simulink model "benchmark_model_2"  (R2021a)
settings: Solver=ode1  StartTime=0.0  StopTime=Tend  FixedStep=0.0001  MaxStep=0.1  MinStep=0.0001  AbsTol=0.01  EnableMultiTasking=on
values from neighbouring files (symbols this model uses):
  A1 = 0.00017774967488    [engine_data.mat]
  A2 = 740220.330082    [engine_data.mat]
  AL = [6 6.5 7 7.5 8 8.5 9 9.5 10 10.5 11 11.5 ... (33 elements, 33x1)]    [engine_data.mat]
  AM0 = 0.02884    [engine_data.mat]
  AREA = 0.00580880481649    [engine_data.mat]
  BORE = 0.086    [engine_data.mat]
  C_EGR = 1.5    [engine_data.mat]
  c_f = 800000    [engine_data.mat]
  c_T = 1    [engine_data.mat]
  CAIR = [0 0 0 0.21 0 0 0.79]    [engine_data.mat]
  cCO = 0    [engine_data.mat]
  cCO2 = 0    [engine_data.mat]
  cH2 = 0    [engine_data.mat]
  cH2O = 0    [engine_data.mat]
  cHC = 0    [engine_data.mat]
  cN2 = 0.79    [engine_data.mat]
  CO = [22.3416398376 20.8398063107 19.3759939408 17.9445472871 16.538827802 15.1528221174 13.7819470707 12.4234138404 11.076283262 9.74128071245 8.42044156849 7.11667724438 ... (33 elements, 33x1)]    [engine_data.mat]
  CO2 = [1.08016197936 1.63070203699 2.20578946805 2.80905596198 3.44329822989 4.11013545224 4.80975559522 5.54078746844 6.30033629562 7.08419123341 7.88717005398 8.70352822078 ... (33 elements, 33x1)]    [engine_data.mat]
  cO2 = 0.21    [engine_data.mat]
  DEN0 = 1.17881164668    [engine_data.mat]
  EGR_dia = 0.02    [engine_data.mat]
  EGR_sk = 0.125663706144    [engine_data.mat]
  EX_AREA = 0.00137444678595    [engine_data.mat]
  EX_M_AR = 0.0258532162804    [engine_data.mat]
  EXO = 40    [engine_data.mat]
  FD0 = 5    [engine_data.mat]
  FOM = [12 11.348 6.233 5 5.449 8.523 5]    [engine_data.mat]
  FR0 = 0    [engine_data.mat]
  FR_C1 = 305.731    [engine_data.mat]
  FR_C2 = 1.70183    [engine_data.mat]
  FR_C3 = 3188.7424    [engine_data.mat]
  FR_C4 = 0.000296028194151    [engine_data.mat]
  FR_C5 = 1.03    [engine_data.mat]
  H2 = [17.3855302766 15.0102176452 12.8820660449 10.9850020715 9.30240027035 7.81790027685 6.51548255669 5.37933989743 4.39378660966 3.5433012035 2.8127075229 2.1874445405 ... (33 elements, 33x1)]    [engine_data.mat]
  H2O = [3.81120036781 5.32559240945 6.64944794012 7.79700886885 8.78142378855 9.61507632366 10.310008356 10.8782622871 11.3320540899 11.6837509075 11.9456809954 12.1298414055 ... (33 elements, 33x1)]    [engine_data.mat]
  HC = [5481.3024964 4476.06435729 3754.34247414 3215.30411383 2799.83726136 2471.30975971 2205.97110777 1987.83348465 1805.78690133 1651.89669698 1520.35918152 1406.8402103 ... (33 elements, 33x1)]    [engine_data.mat]
  INC = 0    [engine_data.mat]
  INO = -40    [engine_data.mat]
  KET = 0.001    [engine_data.mat]
  Kex = 1.28224854645    [engine_data.mat]
  Kh = 0.00462    [engine_data.mat]
  MAS0 = 0.00471524658673    [engine_data.mat]
  MCh = 0.000588883862304    [engine_data.mat]
  MHC = 0.01383448    [engine_data.mat]
  MN2 = 0.028    [engine_data.mat]
  MO2 = 0.032    [engine_data.mat]
  MOLcylT = 0.00157069204711    [engine_data.mat]
  N2 = [54.5020363032 56.4529864816 58.2465252261 59.8999246568 61.4284172656 62.8453054261 64.1621746691 65.3891205654 66.5349581592 67.6074047194 68.6132342687 69.5584035698 ... (33 elements, 33x1)]    [engine_data.mat]
  O2 = [0.331300985803 0.293088680307 0.264743132617 0.242930742419 0.225648917415 0.211629427842 0.200034641439 0.190292592782 0.182002893523 0.174881554044 0.168729672297 0.163420998081 ... (33 elements, 33x1)]    [engine_data.mat]
  PR0 = 101324.72    [engine_data.mat]
  R150 = 157.079632679    [engine_data.mat]
  Rabs = 8.31441    [engine_data.mat]
  SPEC = [4 0.086 0.086 0.043 0.14665 14 1 0.1 0 0.5 0.005 0 ... (19 elements, 19x1)]    [engine_data.mat]
  TBORE = 0.055    [engine_data.mat]
  Tend = 120    [engine_data.mat]
  Th_HC = 0.1    [engine_data.mat]
  Th_knock = 0.401961937891    [engine_data.mat]
  THEX = [0 1 2 3 4 5 6 7 8 9 10 11 ... (721 elements, 1x721)]    [engine_data.mat]
  THIN = [0 1 2 3 4 5 6 7 8 9 10 11 ... (721 elements, 1x721)]    [engine_data.mat]
  TM0 = 298.15    [engine_data.mat]
  Tstart = 5    [engine_data.mat]
  TW0 = 353.15    [engine_data.mat]
  V_EX = 0.0001    [engine_data.mat]
  VAREX = [0 0 0 0 0 0 0 0 0 0 0 0 ... (721 elements, 1x721)]    [engine_data.mat]
  VARIN = [0 0 0 0 0 0 0 0 0 0 0 0 ... (721 elements, 1x721)]    [engine_data.mat]
  VH = 0.000499557214218    [engine_data.mat]
  VT = 3.84274780168e-05    [engine_data.mat]
  WOM = [0.01383448 0.04401 0.02801 0.032 0.002016 0.018016 0.028]    [engine_data.mat]
  y = 1.81    [engine_data.mat]
undefined symbols (not defined in the file or in its folder): DiscIntNeverNeededParam
libraries: pid_lib x3
(part 5 of 7)

== system benchmark_model_2/ENGINE/engine_s/cylinders/cyl3/cyl/knock_Integral/Subsystem1 ==
  pc : Inport
  rps : Inport  Port=2
  Tc : Inport  Port=3
  rad : Inport  Port=4
  Constant1 : Constant  Value=0
  Constant2 : Constant  Value=FR_C1
  Constant3 : Constant
  Constant4 : Constant  Value=(540+INC)*pi/180
  Constant5 : Constant  Value=(180-EXO)*pi/180
  Divide1 : Product  Inputs=3
  Divide2 : Product  Inputs=*/
  Fcn : Fcn  Expr=-FR_C2*(-FR_C4*u+FR_C5)
  Gain : Gain  Gain=0.001
  Integrator : Integrator  ExternalReset=rising
  Math Function : Math  Operator=pow  SignedPower=on  SaturateOnIntegerOverflow=on
  Memory : Memory
  Relational Operator1 : RelationalOperator  Operator=<=  OutDataTypeStr=boolean  RndMeth=Nearest
  Relational Operator2 : RelationalOperator  OutDataTypeStr=boolean  RndMeth=Nearest
  Saturation : Saturate  UpperLimit=inf  LowerLimit=1.0e-16
  Subsystem : Subsystem
  Switch : Switch  Threshold=0.5
  cal_unburned_temp : Subsystem
  ki : Outport
  wires:
  pc/1 -> Saturation/1
  Fcn/1 -> Math Function/2
  Math Function/1 -> Divide1/2
  Constant2/1 -> Divide1/1
  Subsystem/1(Out1) -> Divide1/3
  Divide1/1 -> Divide2/2
  Constant3/1 -> Divide2/1
  Divide2/1 -> Integrator/1
  Tc/1 -> cal_unburned_temp/2(Tc)
  Memory/1 -> Integrator/2
  cal_unburned_temp/1(Tu) -> Subsystem/1(Tu)
  Gain/1 -> Math Function/1
  Integrator/1 -> Switch/1
  Switch/1 -> ki/1
  Constant1/1 -> Switch/3
  rad/1 -> Relational Operator1/1, Relational Operator2/1
  Constant4/1 -> Relational Operator2/2
  Relational Operator2/1 -> cal_unburned_temp/3(trg_inc), Memory/1
  Constant5/1 -> Relational Operator1/2
  Relational Operator1/1 -> Switch/2
  rps/1 -> Fcn/1
  Saturation/1 -> cal_unburned_temp/1(Pc), Gain/1

== system benchmark_model_2/ENGINE/engine_s/cylinders/cyl3/cyl/knock_Integral/Triggered Subsystem ==
  QA_max : Inport
  QA : Inport  Port=2
  Trigger : TriggerPort  VariantControl=(inherit)
  Constant1 : Constant  Value=0
  Constant2 : Constant  Value=1.0e-9
  Relational Operator : RelationalOperator  OutDataTypeStr=boolean  RndMeth=Nearest
  Subtract : Sum  Inputs=+-
  Switch : Switch  Threshold=0.5
  AI_Q : Outport  InitialOutput=0
  wires:
  QA/1 -> Subtract/2
  QA_max/1 -> Subtract/1
  Constant1/1 -> Switch/3
  Switch/1 -> AI_Q/1
  Subtract/1 -> Relational Operator/1, Switch/1
  Relational Operator/1 -> Switch/2
  Constant2/1 -> Relational Operator/2

== system benchmark_model_2/ENGINE/engine_s/cylinders/cyl3/cyl/ramining ratio of fuel/Triggered Subsystem ==
  QA : Inport
  Trigger : TriggerPort  VariantControl=(inherit)
  Constant : Constant
  Constant1 : Constant  Value=0
  Constant2 : Constant  Value=1.0e-9
  Relational Operator : RelationalOperator  OutDataTypeStr=boolean  RndMeth=Nearest
  Subtract : Sum  Inputs=+-
  Switch : Switch  Threshold=0.5
  AI_Q : Outport  InitialOutput=0
  wires:
  Constant2/1 -> Relational Operator/2
  Relational Operator/1 -> Switch/2
  Subtract/1 -> Switch/1, Relational Operator/1
  Switch/1 -> AI_Q/1
  Constant1/1 -> Switch/3
  Constant/1 -> Subtract/1
  QA/1 -> Subtract/2

== system benchmark_model_2/ENGINE/engine_s/cylinders/cyl3/cyl/unburnt_gass/add_fuel1 ==
  Nfuel : Inport
  mol : Inport  Port=2
  Add : Sum
  Demux : Demux  Outputs=7
  Mux : Mux  Inputs=7
  add_fuel : Outport
  wires:
  Demux/2 -> Mux/2
  Demux/3 -> Mux/3
  Demux/4 -> Mux/4
  Demux/5 -> Mux/5
  Demux/6 -> Mux/6
  Demux/7 -> Mux/7
  mol/1 -> Demux/1
  Mux/1 -> add_fuel/1
  Demux/1 -> Add/2
  Add/1 -> Mux/1
  Nfuel/1 -> Add/1

== system benchmark_model_2/ENGINE/engine_s/cylinders/cyl3/cyl/unburnt_gass/init&trig ==
  trig : Inport
  value : Inport  Port=2
  Demux : Demux  Outputs=7
  Mux : Mux  Inputs=7
  qChart : Stateflow chart  TreatAsAtomicUnit=on
  init : Outport
  wires:
  value/1 -> Demux/1
  Demux/1 -> qChart/1(sl_in1)
  Demux/2 -> qChart/2(sl_in2)
  Demux/3 -> qChart/3(sl_in3)
  Demux/4 -> qChart/4(sl_in4)
  Demux/5 -> qChart/5(sl_in5)
  Demux/6 -> qChart/6(sl_in6)
  Demux/7 -> qChart/7(sl_in7)
  qChart/7(sl_out7) -> Mux/7
  qChart/1(sl_out1) -> Mux/1
  qChart/2(sl_out2) -> Mux/2
  qChart/3(sl_out3) -> Mux/3
  qChart/4(sl_out4) -> Mux/4
  qChart/5(sl_out5) -> Mux/5
  qChart/6(sl_out6) -> Mux/6
  Mux/1 -> init/1
  trig/1 -> qChart/Trigger

== system benchmark_model_2/ENGINE/engine_s/cylinders/cyl3/selectors/selector/mod720(u,4*pi) ==
  u : Inport
  Constant7 : Constant  Value=4*pi
  Math Function : Math  Operator=mod  SignedPower=on  SaturateOnIntegerOverflow=on
  y : Outport
  wires:
  Math Function/1 -> y/1
  u/1 -> Math Function/1
  Constant7/1 -> Math Function/2

== system benchmark_model_2/ENGINE/engine_s/cylinders/cyl4/cyl/Energy_Int/dvol ==
  rad : Inport
  rps : Inport  Port=2
  Product : Product  RndMeth=Zero
  func_d_cylvol(u,SPEC) : Subsystem
  dvol : Outport
  wires:
  func_d_cylvol(u,SPEC)/1(Out1) -> Product/1
  rad/1 -> func_d_cylvol(u,SPEC)/1(In1)
  Product/1 -> dvol/1
  rps/1 -> Product/2

== system benchmark_model_2/ENGINE/engine_s/cylinders/cyl4/cyl/cal_cyl_state/cal_state ==
  note: p/d = R T
      | T = P/d/R
  m : Inport
  n : Inport  Port=2
  f : Inport  Port=3
  E : Inport  Port=4
  vol : Inport  Port=5
  Fcn : Fcn  Expr=2/u[1]*u[3]/u[2]
  Fcn1 : Fcn  Expr=u[3]/u[1]/(Rabs/u[2])
  Mux : Mux  Inputs=3
  Mux1 : Mux
  Mux2 : Mux  Inputs=3
  Product1 : Product  Inputs=/*  RndMeth=Zero
  Product2 : Product  Inputs=*/  RndMeth=Zero
  Product3 : Product  Inputs=*/  RndMeth=Zero
  pc : Outport  InitialOutput=0
  tc : Outport  Port=2  InitialOutput=0
  cyl_st : Outport  Port=3  InitialOutput=0
  wires:
  Fcn1/1 -> tc/1
  E/1 -> Mux/3
  f/1 -> Product1/2
  n/1 -> Product2/2, Product1/1
  m/1 -> Product3/1, Product2/1
  Mux2/1 -> Fcn1/1
  Product3/1 -> Mux1/1, Mux2/1  "dens"
  Product2/1 -> Mux1/3, Mux2/2  "gas_c"
  Product1/1 -> Mux1/4, Mux/1  "deg of freedom"
  vol/1 -> Product3/2, Mux/2
  Mux1/1 -> cyl_st/1
  Mux/1 -> Fcn/1
  Fcn/1 -> pc/1, Mux2/3, Mux1/2  "pres"

== system benchmark_model_2/ENGINE/engine_s/cylinders/cyl4/cyl/crank/Subsystem1 ==
  trig_inj : Inport
  fc : Inport  Port=2
  N/s : Inport  Port=3
  Gain : Gain  Gain=MHC
  Integrator : Integrator  ExternalReset=rising
  Product : Product
  Relational Operator1 : RelationalOperator  OutDataTypeStr=boolean  RndMeth=Nearest
  N_fuel : Outport
  wires:
  Gain/1 -> Integrator/1
  N/s/1 -> Gain/1, Product/2
  fc/1 -> Relational Operator1/1
  Relational Operator1/1 -> Product/1
  Integrator/1 -> Relational Operator1/2
  Product/1 -> N_fuel/1
  trig_inj/1 -> Integrator/2

== system benchmark_model_2/ENGINE/engine_s/cylinders/cyl4/cyl/crank/inj_start ==
  rad : Inport
  Constant3 : Constant  Value=(360-INO+1)*pi/180
  Relational Operator2 : RelationalOperator  OutDataTypeStr=boolean  RndMeth=Nearest
  trig_inj : Outport
  wires:
  Relational Operator2/1 -> trig_inj/1
  rad/1 -> Relational Operator2/1
  Constant3/1 -> Relational Operator2/2

== system benchmark_model_2/ENGINE/engine_s/cylinders/cyl4/cyl/crank/mol_flow_rate ==
  rps : Inport
  Constant1 : Constant  Value=0.50*pi
  Constant2 : Constant  Value=MHC
  Divide2 : Product  Inputs=*/
  Divide3 : Product  Inputs=*/
  Divide4 : Product  Inputs=*/
  inje/s : Constant  Value=(DEN0*VH/14.5)
  N/s : Outport
  wires:
  Divide2/1 -> Divide3/1
  Divide4/1 -> Divide2/2
  rps/1 -> Divide4/2
  Constant1/1 -> Divide4/1
  inje/s/1 -> Divide2/1
  Divide3/1 -> N/s/1
  Constant2/1 -> Divide3/2

== system benchmark_model_2/ENGINE/engine_s/cylinders/cyl4/cyl/frame/Init_cyl_gas ==
  tr_inc : Inport
  mol_s : Inport  Port=2
  capture_cyl_state : Subsystem  TreatAsAtomicUnit=on
  init_gas : Outport
  Qmax : Outport  Port=2
  b_comp : Outport  Port=3
  af : Outport  Port=4
  wires:
  tr_inc/1 -> capture_cyl_state/Trigger
  capture_cyl_state/4(af) -> af/1
  capture_cyl_state/1(Qmax) -> Qmax/1
  mol_s/1 -> capture_cyl_state/1(cyl_gas)
  capture_cyl_state/2(b_comp) -> b_comp/1
  capture_cyl_state/3(init_gas) -> init_gas/1

== system benchmark_model_2/ENGINE/engine_s/cylinders/cyl4/cyl/frame/ratio_burnt1 ==
  rps : Inport
  rad : Inport  Port=2
  AF : Inport  Port=3
  KL : Inport  Port=4
  SA : Inport  Port=5
  EGR : Inport  Port=6
  VT : Inport  Port=7
  Add : Sum
  Constant : Constant  Value=(180-EXO-1)*pi/180+pi
  Constant1 : Constant  Value=0
  Constant2 : Constant  Value=pi
  Constant3 : Constant  Value=0
  Product : Product  RndMeth=Zero
  Relational Operator : RelationalOperator  Operator=<  OutDataTypeStr=boolean  RndMeth=Nearest
  Switch : Switch  Threshold=0.5
  Switch1 : Switch  Threshold=0.5
  mod720(u,4*pi) : Subsystem
  murnt_ratio : Subsystem
  burnt_ratio : Outport  PortDimensions=1  InitialOutput=0
  QR : Outport  Port=2  PortDimensions=1  InitialOutput=0
  Q : Outport  Port=3  PortDimensions=1  InitialOutput=0
  wires:
  VT/1 -> murnt_ratio/7(VT)
  Switch1/1 -> Q/1
  Constant3/1 -> Switch1/3
  murnt_ratio/2(Q) -> Switch1/1
  Constant2/1 -> Add/1
  rad/1 -> Add/2
  Add/1 -> mod720(u,4*pi)/1(u)
  EGR/1 -> murnt_ratio/6(EGR)
  Product/1 -> burnt_ratio/1
  Switch/1 -> QR/1, Product/1
  Constant1/1 -> Switch/3
  Relational Operator/1 -> Switch/2, Switch1/2
  Constant/1 -> Relational Operator/2
  SA/1 -> murnt_ratio/2(SA)
  KL/1 -> murnt_ratio/4(KL)
  AF/1 -> murnt_ratio/5(AF)
  rps/1 -> Product/2, murnt_ratio/3(rps)
  mod720(u,4*pi)/1(y) -> Relational Operator/1, murnt_ratio/1(u)
  murnt_ratio/1(q) -> Switch/1

== system benchmark_model_2/ENGINE/engine_s/cylinders/cyl4/cyl/heat_trans/cal_cyl_ar ==
  vol : Inport
  Add2 : Sum
  Constant1 : Constant  Value=2*pi*BORE
  Constant2 : Constant  Value=AREA
  Gain1 : Gain  Gain=2
  Product1 : Product  Inputs=*/  RndMeth=Zero
  Product2 : Product  RndMeth=Zero
  cyl_ar : Outport
  wires:
  Product2/1 -> Add2/1
  Constant1/1 -> Product2/1
  Product1/1 -> Product2/2
  Add2/1 -> cyl_ar/1
  vol/1 -> Product1/1
  Gain1/1 -> Add2/2
  Constant2/1 -> Gain1/1, Product1/2

== system benchmark_model_2/ENGINE/engine_s/cylinders/cyl4/cyl/heat_trans/cal_qw ==
  pc : Inport
  rps : Inport  Port=2
  Tg : Inport  Port=3
  Tw : Inport  Port=4
  Fcn : Fcn  Expr=(u(1)*u(2))^0.786*u(3)^(-0.525)*(u(3)-u(4))
  Mux3 : Mux
  Saturation : Saturate  UpperLimit=inf  LowerLimit=1.0e-16
  qw : Outport
  wires:
  Saturation/1 -> Fcn/1
  Tg/1 -> Mux3/3
  rps/1 -> Mux3/2
  pc/1 -> Mux3/1
  Tw/1 -> Mux3/4
  Fcn/1 -> qw/1
  Mux3/1 -> Saturation/1

== system benchmark_model_2/ENGINE/engine_s/cylinders/cyl4/cyl/heat_trans/cyl_wall ==
  qw_v : Inport
  Tw0 : Inport  Port=2
  Gain1 : Gain  Gain=1/2.5
  Gain2 : Gain  Gain=1.0
  Gain5 : Gain  Gain=3.0
  Integrator : Integrator  InitialConditionSource=external
  Subtract : Sum  Inputs=-+
  Subtract2 : Sum  Inputs=+-
  Tw : Outport
  wires:
  qw_v/1 -> Gain2/1
  Gain5/1 -> Subtract/1
  Subtract2/1 -> Gain5/1
  Gain2/1 -> Subtract/2
  Integrator/1 -> Subtract2/1, Tw/1
  Gain1/1 -> Integrator/1
  Subtract/1 -> Gain1/1
  Tw0/1 -> Integrator/2, Subtract2/2

== system benchmark_model_2/ENGINE/engine_s/cylinders/cyl4/cyl/knock_Integral/Subsystem1 ==
  pc : Inport
  rps : Inport  Port=2
  Tc : Inport  Port=3
  rad : Inport  Port=4
  Constant1 : Constant  Value=0
  Constant2 : Constant  Value=FR_C1
  Constant3 : Constant
  Constant4 : Constant  Value=(540+INC)*pi/180
  Constant5 : Constant  Value=(180-EXO)*pi/180
  Divide1 : Product  Inputs=3
  Divide2 : Product  Inputs=*/
  Fcn : Fcn  Expr=-FR_C2*(-FR_C4*u+FR_C5)
  Gain : Gain  Gain=0.001
  Integrator : Integrator  ExternalReset=rising
  Math Function : Math  Operator=pow  SignedPower=on  SaturateOnIntegerOverflow=on
  Memory : Memory
  Relational Operator1 : RelationalOperator  Operator=<=  OutDataTypeStr=boolean  RndMeth=Nearest
  Relational Operator2 : RelationalOperator  OutDataTypeStr=boolean  RndMeth=Nearest
  Saturation : Saturate  UpperLimit=inf  LowerLimit=1.0e-16
  Subsystem : Subsystem
  Switch : Switch  Threshold=0.5
  cal_unburned_temp : Subsystem
  ki : Outport
  wires:
  Saturation/1 -> Gain/1, cal_unburned_temp/1(Pc)
  rps/1 -> Fcn/1
  Relational Operator1/1 -> Switch/2
  Constant5/1 -> Relational Operator1/2
  Relational Operator2/1 -> Memory/1, cal_unburned_temp/3(trg_inc)
  Constant4/1 -> Relational Operator2/2
  rad/1 -> Relational Operator2/1, Relational Operator1/1
  Constant1/1 -> Switch/3
  Switch/1 -> ki/1
  Integrator/1 -> Switch/1
  Gain/1 -> Math Function/1
  cal_unburned_temp/1(Tu) -> Subsystem/1(Tu)
  Memory/1 -> Integrator/2
  Tc/1 -> cal_unburned_temp/2(Tc)
  Divide2/1 -> Integrator/1
  Constant3/1 -> Divide2/1
  Divide1/1 -> Divide2/2
  Subsystem/1(Out1) -> Divide1/3
  Constant2/1 -> Divide1/1
  Math Function/1 -> Divide1/2
  Fcn/1 -> Math Function/2
  pc/1 -> Saturation/1

== system benchmark_model_2/ENGINE/engine_s/cylinders/cyl4/cyl/knock_Integral/Triggered Subsystem ==
  QA_max : Inport
  QA : Inport  Port=2
  Trigger : TriggerPort  VariantControl=(inherit)
  Constant1 : Constant  Value=0
  Constant2 : Constant  Value=1.0e-9
  Relational Operator : RelationalOperator  OutDataTypeStr=boolean  RndMeth=Nearest
  Subtract : Sum  Inputs=+-
  Switch : Switch  Threshold=0.5
  AI_Q : Outport  InitialOutput=0
  wires:
  Constant2/1 -> Relational Operator/2
  Relational Operator/1 -> Switch/2
  Subtract/1 -> Switch/1, Relational Operator/1
  Switch/1 -> AI_Q/1
  Constant1/1 -> Switch/3
  QA_max/1 -> Subtract/1
  QA/1 -> Subtract/2

== system benchmark_model_2/ENGINE/engine_s/cylinders/cyl4/cyl/ramining ratio of fuel/Triggered Subsystem ==
  QA : Inport
  Trigger : TriggerPort  VariantControl=(inherit)
  Constant : Constant
  Constant1 : Constant  Value=0
  Constant2 : Constant  Value=1.0e-9
  Relational Operator : RelationalOperator  OutDataTypeStr=boolean  RndMeth=Nearest
  Subtract : Sum  Inputs=+-
  Switch : Switch  Threshold=0.5
  AI_Q : Outport  InitialOutput=0
  wires:
  QA/1 -> Subtract/2
  Constant/1 -> Subtract/1
  Constant1/1 -> Switch/3
  Switch/1 -> AI_Q/1
  Subtract/1 -> Relational Operator/1, Switch/1
  Relational Operator/1 -> Switch/2
  Constant2/1 -> Relational Operator/2

== system benchmark_model_2/ENGINE/engine_s/cylinders/cyl4/cyl/unburnt_gass/add_fuel1 ==
  Nfuel : Inport
  mol : Inport  Port=2
  Add : Sum
  Demux : Demux  Outputs=7
  Mux : Mux  Inputs=7
  add_fuel : Outport
  wires:
  Nfuel/1 -> Add/1
  Add/1 -> Mux/1
  Demux/1 -> Add/2
  Mux/1 -> add_fuel/1
  mol/1 -> Demux/1
  Demux/7 -> Mux/7
  Demux/6 -> Mux/6
  Demux/5 -> Mux/5
  Demux/4 -> Mux/4
  Demux/3 -> Mux/3
  Demux/2 -> Mux/2

== system benchmark_model_2/ENGINE/engine_s/cylinders/cyl4/cyl/unburnt_gass/init&trig ==
  trig : Inport
  value : Inport  Port=2
  Demux : Demux  Outputs=7
  Mux : Mux  Inputs=7
  qChart : Stateflow chart  TreatAsAtomicUnit=on
  init : Outport
  wires:
  trig/1 -> qChart/Trigger
  Mux/1 -> init/1
  qChart/6(sl_out6) -> Mux/6
  qChart/5(sl_out5) -> Mux/5
  qChart/4(sl_out4) -> Mux/4
  qChart/3(sl_out3) -> Mux/3
  qChart/2(sl_out2) -> Mux/2
  qChart/1(sl_out1) -> Mux/1
  qChart/7(sl_out7) -> Mux/7
  Demux/7 -> qChart/7(sl_in7)
  Demux/6 -> qChart/6(sl_in6)
  Demux/5 -> qChart/5(sl_in5)
  Demux/4 -> qChart/4(sl_in4)
  Demux/3 -> qChart/3(sl_in3)
  Demux/2 -> qChart/2(sl_in2)
  Demux/1 -> qChart/1(sl_in1)
  value/1 -> Demux/1

== system benchmark_model_2/ENGINE/engine_s/cylinders/cyl4/selectors/selector/mod720(u,4*pi) ==
  u : Inport
  Constant7 : Constant  Value=4*pi
  Math Function : Math  Operator=mod  SignedPower=on  SaturateOnIntegerOverflow=on
  y : Outport
  wires:
  Constant7/1 -> Math Function/2
  u/1 -> Math Function/1
  Math Function/1 -> y/1

== system benchmark_model_2/ENGINE/engine_s/cylinders/cyl1/cyl/Energy_Int/dvol/func_d_cylvol(u,SPEC) ==
  In1 : Inport
  Constant1 : Constant  Value=SPEC
  Embedded MATLAB Function1 : MATLAB Function  TreatAsAtomicUnit=on
  Out1 : Outport
  wires:
  Constant1/1 -> Embedded MATLAB Function1/2(SPEC)
  In1/1 -> Embedded MATLAB Function1/1(u)
  Embedded MATLAB Function1/1(y) -> Out1/1

== system benchmark_model_2/ENGINE/engine_s/cylinders/cyl1/cyl/frame/Init_cyl_gas/capture_cyl_state ==
  cyl_gas : Inport
  Trigger : TriggerPort  VariantControl=(inherit)
  Add : Sum  Inputs=++++
  C+O2->CO2 : Constant  Value=4.19*97200.0
  CO+1/2O2->CO2 : Constant  Value=4.19*29620.0
  H+1/2O2->H2O : Constant  Value=4.19*57750.0
  H+1/2O2->H2O1 : Constant  Value=4.19*57750.0
  H/C : Constant  Value=y/2
  Product : Product  RndMeth=Zero
  Product1 : Product  RndMeth=Zero
  Product2 : Product  RndMeth=Zero
  Product3 : Product  Inputs=3  RndMeth=Zero
  Saturation : Saturate  UpperLimit=22  LowerLimit=6
  Selector1 : Selector  InputPortWidth=7  IndexOptions=Index vector (dialog)  Indices=[3]  OutputSizes=[(-2)]
  Selector2 : Selector  InputPortWidth=7  IndexOptions=Index vector (dialog)  Indices=[5]  OutputSizes=[(-2)]
  Selector3 : Selector  InputPortWidth=7  IndexOptions=Index vector (dialog)  Indices=[1]  OutputSizes=[(-2)]
  Selector4 : Selector  InputPortWidth=7  IndexOptions=Index vector (dialog)  Indices=[1]  OutputSizes=[(-2)]
  Subtract : Sum  Inputs=-+
  burnt_compsition : Subsystem
  cal_af : Subsystem
  Qmax : Outport
  b_comp : Outport  Port=2  InitialOutput=[0;0;0;0;0;0;0]
  init_gas : Outport  Port=3  InitialOutput=[0;0;0;0;0;0;0]
  af : Outport  Port=4  InitialOutput=0
  wires:
  Subtract/1 -> Selector3/1, Selector2/1, Selector1/1, Selector4/1
  Add/1 -> Qmax/1
  H+1/2O2->H2O/1 -> Product2/2
  Selector2/1 -> Product2/1
  CO+1/2O2->CO2/1 -> Product1/2
  Selector1/1 -> Product1/1
  C+O2->CO2/1 -> Product/2
  burnt_compsition/1(b_comp) -> b_comp/1, Subtract/1
  cal_af/1(af) -> Saturation/1, burnt_compsition/1(af)
  cyl_gas/1 -> init_gas/1, burnt_compsition/2(mol_su), Subtract/2, cal_af/1(cyl_gas)
  Product/1 -> Add/1
  Product1/1 -> Add/2
  Product2/1 -> Add/3
  H+1/2O2->H2O1/1 -> Product3/2
  Selector3/1 -> Product3/1
  Product3/1 -> Add/4
  H/C/1 -> Product3/3
  Saturation/1 -> af/1
  Selector4/1 -> Product/1

== system benchmark_model_2/ENGINE/engine_s/cylinders/cyl1/cyl/frame/ratio_burnt1/mod720(u,4*pi) ==
  u : Inport
  Constant7 : Constant  Value=4*pi
  Math Function : Math  Operator=mod  SignedPower=on  SaturateOnIntegerOverflow=on
  y : Outport
  wires:
  Math Function/1 -> y/1
  u/1 -> Math Function/1
  Constant7/1 -> Math Function/2

== system benchmark_model_2/ENGINE/engine_s/cylinders/cyl1/cyl/frame/ratio_burnt1/murnt_ratio ==
  u : Inport
  SA : Inport  Port=2
  rps : Inport  Port=3
  KL : Inport  Port=4
  AF : Inport  Port=5
  EGR : Inport  Port=6
  VT : Inport  Port=7
  Constant2 : Constant  Value=2
  Constant6 : Constant  Value=6
  Embedded MATLAB Function : MATLAB Function  TreatAsAtomicUnit=on
  Gain1 : Gain  Gain=2
  Gain2 : Gain  Gain=180/pi
  Gain3 : Gain  Gain=pi/180
  Mux : Mux
  Phi050 DoE model : Subsystem
  q : Outport
  Q : Outport  Port=2
  wires:
  Gain3/1 -> Mux/4
  Embedded MATLAB Function/1(q) -> q/1
  SA/1 -> Gain3/1, Phi050 DoE model/3(SA)
  Mux/1 -> Embedded MATLAB Function/2(Web)
  Constant6/1 -> Mux/1
  Constant2/1 -> Mux/2
  Phi050 DoE model/1(Phi50) -> Gain1/1
  rps/1 -> Phi050 DoE model/1(N)
  KL/1 -> Phi050 DoE model/2(KL)
  VT/1 -> Gain2/1
  AF/1 -> Phi050 DoE model/5(AFR)
  Gain1/1 -> Mux/3
  EGR/1 -> Phi050 DoE model/6(EGR)
  u/1 -> Embedded MATLAB Function/1(u)
  Embedded MATLAB Function/2(Q) -> Q/1
  Gain2/1 -> Phi050 DoE model/4(VVT)

== system benchmark_model_2/ENGINE/engine_s/cylinders/cyl1/cyl/knock_Integral/Subsystem1/Subsystem ==
  Tu : Inport
  Constant1 : Constant  Value=FR_C3
  Divide : Product  Inputs=/*
  Math Function1 : Math  SignedPower=on  SaturateOnIntegerOverflow=on
  Saturation : Saturate  UpperLimit=inf  LowerLimit=1.0e-5
  Out1 : Outport
  wires:
  Constant1/1 -> Divide/2
  Divide/1 -> Math Function1/1
  Math Function1/1 -> Out1/1
  Tu/1 -> Saturation/1
  Saturation/1 -> Divide/1

== system benchmark_model_2/ENGINE/engine_s/cylinders/cyl1/cyl/knock_Integral/Subsystem1/cal_unburned_temp ==
  Pc : Inport
  Tc : Inport  Port=2
  trg_inc : Inport  Port=3
  Constant : Constant  Value=1-1/Kex
  Divide3 : Product  Inputs=*/
  Divide4 : Product
  Math Function2 : Math  Operator=pow  SignedPower=on  SaturateOnIntegerOverflow=on
  Subsystem : Subsystem
  Tu : Outport
  wires:
  Subsystem/1(Pc_inc) -> Divide3/2
  Divide3/1 -> Math Function2/1
  Math Function2/1 -> Divide4/1
  Subsystem/2(Tc_inc) -> Divide4/2
  Constant/1 -> Math Function2/2
  Divide4/1 -> Tu/1
  Tc/1 -> Subsystem/2(Tc)
  Pc/1 -> Subsystem/1(Pc), Divide3/1
  trg_inc/1 -> Subsystem/Trigger

== system benchmark_model_2/ENGINE/engine_s/cylinders/cyl2/cyl/Energy_Int/dvol/func_d_cylvol(u,SPEC) ==
  In1 : Inport
  Constant1 : Constant  Value=SPEC
  Embedded MATLAB Function1 : MATLAB Function  TreatAsAtomicUnit=on
  Out1 : Outport
  wires:
  Embedded MATLAB Function1/1(y) -> Out1/1
  In1/1 -> Embedded MATLAB Function1/1(u)
  Constant1/1 -> Embedded MATLAB Function1/2(SPEC)

== system benchmark_model_2/ENGINE/engine_s/cylinders/cyl2/cyl/frame/Init_cyl_gas/capture_cyl_state ==
  cyl_gas : Inport
  Trigger : TriggerPort  VariantControl=(inherit)
  Add : Sum  Inputs=++++
  C+O2->CO2 : Constant  Value=4.19*97200.0
  CO+1/2O2->CO2 : Constant  Value=4.19*29620.0
  H+1/2O2->H2O : Constant  Value=4.19*57750.0
  H+1/2O2->H2O1 : Constant  Value=4.19*57750.0
  H/C : Constant  Value=y/2
  Product : Product  RndMeth=Zero
  Product1 : Product  RndMeth=Zero
  Product2 : Product  RndMeth=Zero
  Product3 : Product  Inputs=3  RndMeth=Zero
  Saturation : Saturate  UpperLimit=22  LowerLimit=6
  Selector1 : Selector  InputPortWidth=7  IndexOptions=Index vector (dialog)  Indices=[3]  OutputSizes=[(-2)]
  Selector2 : Selector  InputPortWidth=7  IndexOptions=Index vector (dialog)  Indices=[5]  OutputSizes=[(-2)]
  Selector3 : Selector  InputPortWidth=7  IndexOptions=Index vector (dialog)  Indices=[1]  OutputSizes=[(-2)]
  Selector4 : Selector  InputPortWidth=7  IndexOptions=Index vector (dialog)  Indices=[1]  OutputSizes=[(-2)]
  Subtract : Sum  Inputs=-+
  burnt_compsition : Subsystem
  cal_af : Subsystem
  Qmax : Outport
  b_comp : Outport  Port=2  InitialOutput=[0;0;0;0;0;0;0]
  init_gas : Outport  Port=3  InitialOutput=[0;0;0;0;0;0;0]
  af : Outport  Port=4  InitialOutput=0
  wires:
  Selector4/1 -> Product/1
  Saturation/1 -> af/1
  H/C/1 -> Product3/3
  Product3/1 -> Add/4
  Selector3/1 -> Product3/1
  H+1/2O2->H2O1/1 -> Product3/2
  Product2/1 -> Add/3
  Product1/1 -> Add/2
  Product/1 -> Add/1
  cyl_gas/1 -> cal_af/1(cyl_gas), Subtract/2, burnt_compsition/2(mol_su), init_gas/1
  cal_af/1(af) -> burnt_compsition/1(af), Saturation/1
  burnt_compsition/1(b_comp) -> Subtract/1, b_comp/1
  C+O2->CO2/1 -> Product/2
  Selector1/1 -> Product1/1
  CO+1/2O2->CO2/1 -> Product1/2
  Selector2/1 -> Product2/1
  H+1/2O2->H2O/1 -> Product2/2
  Add/1 -> Qmax/1
  Subtract/1 -> Selector4/1, Selector1/1, Selector2/1, Selector3/1

== system benchmark_model_2/ENGINE/engine_s/cylinders/cyl2/cyl/frame/ratio_burnt1/mod720(u,4*pi) ==
  u : Inport
  Constant7 : Constant  Value=4*pi
  Math Function : Math  Operator=mod  SignedPower=on  SaturateOnIntegerOverflow=on
  y : Outport
  wires:
  Constant7/1 -> Math Function/2
  u/1 -> Math Function/1
  Math Function/1 -> y/1

== system benchmark_model_2/ENGINE/engine_s/cylinders/cyl2/cyl/frame/ratio_burnt1/murnt_ratio ==
  u : Inport
  SA : Inport  Port=2
  rps : Inport  Port=3
  KL : Inport  Port=4
  AF : Inport  Port=5
  EGR : Inport  Port=6
  VT : Inport  Port=7
  Constant2 : Constant  Value=2
  Constant6 : Constant  Value=6
  Embedded MATLAB Function : MATLAB Function  TreatAsAtomicUnit=on
  Gain1 : Gain  Gain=2
  Gain2 : Gain  Gain=180/pi
  Gain3 : Gain  Gain=pi/180
  Mux : Mux
  Phi050 DoE model : Subsystem
  q : Outport
  Q : Outport  Port=2
  wires:
  Gain2/1 -> Phi050 DoE model/4(VVT)
  Embedded MATLAB Function/2(Q) -> Q/1
  u/1 -> Embedded MATLAB Function/1(u)
  EGR/1 -> Phi050 DoE model/6(EGR)
  Gain1/1 -> Mux/3
  AF/1 -> Phi050 DoE model/5(AFR)
  VT/1 -> Gain2/1
  KL/1 -> Phi050 DoE model/2(KL)
  rps/1 -> Phi050 DoE model/1(N)
  Phi050 DoE model/1(Phi50) -> Gain1/1
  Constant2/1 -> Mux/2
  Constant6/1 -> Mux/1
  Mux/1 -> Embedded MATLAB Function/2(Web)
  SA/1 -> Phi050 DoE model/3(SA), Gain3/1
  Embedded MATLAB Function/1(q) -> q/1
  Gain3/1 -> Mux/4

== system benchmark_model_2/ENGINE/engine_s/cylinders/cyl2/cyl/knock_Integral/Subsystem1/Subsystem ==
  Tu : Inport
  Constant1 : Constant  Value=FR_C3
  Divide : Product  Inputs=/*
  Math Function1 : Math  SignedPower=on  SaturateOnIntegerOverflow=on
  Saturation : Saturate  UpperLimit=inf  LowerLimit=1.0e-5
  Out1 : Outport
  wires:
  Saturation/1 -> Divide/1
  Tu/1 -> Saturation/1
  Math Function1/1 -> Out1/1
  Divide/1 -> Math Function1/1
  Constant1/1 -> Divide/2

== system benchmark_model_2/ENGINE/engine_s/cylinders/cyl2/cyl/knock_Integral/Subsystem1/cal_unburned_temp ==
  Pc : Inport
  Tc : Inport  Port=2
  trg_inc : Inport  Port=3
  Constant : Constant  Value=1-1/Kex
  Divide3 : Product  Inputs=*/
  Divide4 : Product
  Math Function2 : Math  Operator=pow  SignedPower=on  SaturateOnIntegerOverflow=on
  Subsystem : Subsystem
  Tu : Outport
  wires:
  trg_inc/1 -> Subsystem/Trigger
  Pc/1 -> Divide3/1, Subsystem/1(Pc)
  Tc/1 -> Subsystem/2(Tc)
  Divide4/1 -> Tu/1
  Constant/1 -> Math Function2/2
  Subsystem/2(Tc_inc) -> Divide4/2
  Math Function2/1 -> Divide4/1
  Divide3/1 -> Math Function2/1
  Subsystem/1(Pc_inc) -> Divide3/2

== system benchmark_model_2/ENGINE/engine_s/cylinders/cyl3/cyl/Energy_Int/dvol/func_d_cylvol(u,SPEC) ==
  In1 : Inport
  Constant1 : Constant  Value=SPEC
  Embedded MATLAB Function1 : MATLAB Function  TreatAsAtomicUnit=on
  Out1 : Outport
  wires:
  Constant1/1 -> Embedded MATLAB Function1/2(SPEC)
  In1/1 -> Embedded MATLAB Function1/1(u)
  Embedded MATLAB Function1/1(y) -> Out1/1

== system benchmark_model_2/ENGINE/engine_s/cylinders/cyl3/cyl/frame/Init_cyl_gas/capture_cyl_state ==
  cyl_gas : Inport
  Trigger : TriggerPort  VariantControl=(inherit)
  Add : Sum  Inputs=++++
  C+O2->CO2 : Constant  Value=4.19*97200.0
  CO+1/2O2->CO2 : Constant  Value=4.19*29620.0
  H+1/2O2->H2O : Constant  Value=4.19*57750.0
  H+1/2O2->H2O1 : Constant  Value=4.19*57750.0
  H/C : Constant  Value=y/2
  Product : Product  RndMeth=Zero
  Product1 : Product  RndMeth=Zero
  Product2 : Product  RndMeth=Zero
  Product3 : Product  Inputs=3  RndMeth=Zero
  Saturation : Saturate  UpperLimit=22  LowerLimit=6
  Selector1 : Selector  InputPortWidth=7  IndexOptions=Index vector (dialog)  Indices=[3]  OutputSizes=[(-2)]
  Selector2 : Selector  InputPortWidth=7  IndexOptions=Index vector (dialog)  Indices=[5]  OutputSizes=[(-2)]
  Selector3 : Selector  InputPortWidth=7  IndexOptions=Index vector (dialog)  Indices=[1]  OutputSizes=[(-2)]
  Selector4 : Selector  InputPortWidth=7  IndexOptions=Index vector (dialog)  Indices=[1]  OutputSizes=[(-2)]
  Subtract : Sum  Inputs=-+
  burnt_compsition : Subsystem
  cal_af : Subsystem
  Qmax : Outport
  b_comp : Outport  Port=2  InitialOutput=[0;0;0;0;0;0;0]
  init_gas : Outport  Port=3  InitialOutput=[0;0;0;0;0;0;0]
  af : Outport  Port=4  InitialOutput=0
  wires:
  Subtract/1 -> Selector3/1, Selector2/1, Selector1/1, Selector4/1
  Add/1 -> Qmax/1
  H+1/2O2->H2O/1 -> Product2/2
  Selector2/1 -> Product2/1
  CO+1/2O2->CO2/1 -> Product1/2
  Selector1/1 -> Product1/1
  C+O2->CO2/1 -> Product/2
  burnt_compsition/1(b_comp) -> b_comp/1, Subtract/1
  cal_af/1(af) -> Saturation/1, burnt_compsition/1(af)
  cyl_gas/1 -> init_gas/1, burnt_compsition/2(mol_su), Subtract/2, cal_af/1(cyl_gas)
  Product/1 -> Add/1
  Product1/1 -> Add/2
  Product2/1 -> Add/3
  H+1/2O2->H2O1/1 -> Product3/2
  Selector3/1 -> Product3/1
  Product3/1 -> Add/4
  H/C/1 -> Product3/3
  Saturation/1 -> af/1
  Selector4/1 -> Product/1

== system benchmark_model_2/ENGINE/engine_s/cylinders/cyl3/cyl/frame/ratio_burnt1/mod720(u,4*pi) ==
  u : Inport
  Constant7 : Constant  Value=4*pi
  Math Function : Math  Operator=mod  SignedPower=on  SaturateOnIntegerOverflow=on
  y : Outport
  wires:
  Math Function/1 -> y/1
  u/1 -> Math Function/1
  Constant7/1 -> Math Function/2

== system benchmark_model_2/ENGINE/engine_s/cylinders/cyl3/cyl/frame/ratio_burnt1/murnt_ratio ==
  u : Inport
  SA : Inport  Port=2
  rps : Inport  Port=3
  KL : Inport  Port=4
  AF : Inport  Port=5
  EGR : Inport  Port=6
  VT : Inport  Port=7
  Constant2 : Constant  Value=2
  Constant6 : Constant  Value=6
  Embedded MATLAB Function : MATLAB Function  TreatAsAtomicUnit=on
  Gain1 : Gain  Gain=2
  Gain2 : Gain  Gain=180/pi
  Gain3 : Gain  Gain=pi/180
  Mux : Mux
  Phi050 DoE model : Subsystem
  q : Outport
  Q : Outport  Port=2
  wires:
  Gain3/1 -> Mux/4
  Embedded MATLAB Function/1(q) -> q/1
  SA/1 -> Gain3/1, Phi050 DoE model/3(SA)
  Mux/1 -> Embedded MATLAB Function/2(Web)
  Constant6/1 -> Mux/1
  Constant2/1 -> Mux/2
  Phi050 DoE model/1(Phi50) -> Gain1/1
  rps/1 -> Phi050 DoE model/1(N)
  KL/1 -> Phi050 DoE model/2(KL)
  VT/1 -> Gain2/1
  AF/1 -> Phi050 DoE model/5(AFR)
  Gain1/1 -> Mux/3
  EGR/1 -> Phi050 DoE model/6(EGR)
  u/1 -> Embedded MATLAB Function/1(u)
  Embedded MATLAB Function/2(Q) -> Q/1
  Gain2/1 -> Phi050 DoE model/4(VVT)

== system benchmark_model_2/ENGINE/engine_s/cylinders/cyl3/cyl/knock_Integral/Subsystem1/Subsystem ==
  Tu : Inport
  Constant1 : Constant  Value=FR_C3
  Divide : Product  Inputs=/*
  Math Function1 : Math  SignedPower=on  SaturateOnIntegerOverflow=on
  Saturation : Saturate  UpperLimit=inf  LowerLimit=1.0e-5
  Out1 : Outport
  wires:
  Constant1/1 -> Divide/2
  Divide/1 -> Math Function1/1
  Math Function1/1 -> Out1/1
  Tu/1 -> Saturation/1
  Saturation/1 -> Divide/1

== system benchmark_model_2/ENGINE/engine_s/cylinders/cyl3/cyl/knock_Integral/Subsystem1/cal_unburned_temp ==
  Pc : Inport
  Tc : Inport  Port=2
  trg_inc : Inport  Port=3
  Constant : Constant  Value=1-1/Kex
  Divide3 : Product  Inputs=*/
  Divide4 : Product
  Math Function2 : Math  Operator=pow  SignedPower=on  SaturateOnIntegerOverflow=on
  Subsystem : Subsystem
  Tu : Outport
  wires:
  Subsystem/1(Pc_inc) -> Divide3/2
  Divide3/1 -> Math Function2/1
  Math Function2/1 -> Divide4/1
  Subsystem/2(Tc_inc) -> Divide4/2
  Constant/1 -> Math Function2/2
  Divide4/1 -> Tu/1
  Tc/1 -> Subsystem/2(Tc)
  Pc/1 -> Subsystem/1(Pc), Divide3/1
  trg_inc/1 -> Subsystem/Trigger

== system benchmark_model_2/ENGINE/engine_s/cylinders/cyl4/cyl/Energy_Int/dvol/func_d_cylvol(u,SPEC) ==
  In1 : Inport
  Constant1 : Constant  Value=SPEC
  Embedded MATLAB Function1 : MATLAB Function  TreatAsAtomicUnit=on
  Out1 : Outport
  wires:
  Embedded MATLAB Function1/1(y) -> Out1/1
  In1/1 -> Embedded MATLAB Function1/1(u)
  Constant1/1 -> Embedded MATLAB Function1/2(SPEC)

== system benchmark_model_2/ENGINE/engine_s/cylinders/cyl4/cyl/frame/Init_cyl_gas/capture_cyl_state ==
  cyl_gas : Inport
  Trigger : TriggerPort  VariantControl=(inherit)
  Add : Sum  Inputs=++++
  C+O2->CO2 : Constant  Value=4.19*97200.0
  CO+1/2O2->CO2 : Constant  Value=4.19*29620.0
  H+1/2O2->H2O : Constant  Value=4.19*57750.0
  H+1/2O2->H2O1 : Constant  Value=4.19*57750.0
  H/C : Constant  Value=y/2
  Product : Product  RndMeth=Zero
  Product1 : Product  RndMeth=Zero
  Product2 : Product  RndMeth=Zero
  Product3 : Product  Inputs=3  RndMeth=Zero
  Saturation : Saturate  UpperLimit=22  LowerLimit=6
  Selector1 : Selector  InputPortWidth=7  IndexOptions=Index vector (dialog)  Indices=[3]  OutputSizes=[(-2)]
  Selector2 : Selector  InputPortWidth=7  IndexOptions=Index vector (dialog)  Indices=[5]  OutputSizes=[(-2)]
  Selector3 : Selector  InputPortWidth=7  IndexOptions=Index vector (dialog)  Indices=[1]  OutputSizes=[(-2)]
  Selector4 : Selector  InputPortWidth=7  IndexOptions=Index vector (dialog)  Indices=[1]  OutputSizes=[(-2)]
  Subtract : Sum  Inputs=-+
  burnt_compsition : Subsystem
  cal_af : Subsystem
  Qmax : Outport
  b_comp : Outport  Port=2  InitialOutput=[0;0;0;0;0;0;0]
  init_gas : Outport  Port=3  InitialOutput=[0;0;0;0;0;0;0]
  af : Outport  Port=4  InitialOutput=0
  wires:
  Selector4/1 -> Product/1
  Saturation/1 -> af/1
  H/C/1 -> Product3/3
  Product3/1 -> Add/4
  Selector3/1 -> Product3/1
  H+1/2O2->H2O1/1 -> Product3/2
  Product2/1 -> Add/3
  Product1/1 -> Add/2
  Product/1 -> Add/1
  cyl_gas/1 -> cal_af/1(cyl_gas), Subtract/2, burnt_compsition/2(mol_su), init_gas/1
  cal_af/1(af) -> burnt_compsition/1(af), Saturation/1
  burnt_compsition/1(b_comp) -> Subtract/1, b_comp/1
  C+O2->CO2/1 -> Product/2
  Selector1/1 -> Product1/1
  CO+1/2O2->CO2/1 -> Product1/2
  Selector2/1 -> Product2/1
  H+1/2O2->H2O/1 -> Product2/2
  Add/1 -> Qmax/1
  Subtract/1 -> Selector4/1, Selector1/1, Selector2/1, Selector3/1

== system benchmark_model_2/ENGINE/engine_s/cylinders/cyl4/cyl/frame/ratio_burnt1/mod720(u,4*pi) ==
  u : Inport
  Constant7 : Constant  Value=4*pi
  Math Function : Math  Operator=mod  SignedPower=on  SaturateOnIntegerOverflow=on
  y : Outport
  wires:
  Constant7/1 -> Math Function/2
  u/1 -> Math Function/1
  Math Function/1 -> y/1

== system benchmark_model_2/ENGINE/engine_s/cylinders/cyl4/cyl/frame/ratio_burnt1/murnt_ratio ==
  u : Inport
  SA : Inport  Port=2
  rps : Inport  Port=3
  KL : Inport  Port=4
  AF : Inport  Port=5
  EGR : Inport  Port=6
  VT : Inport  Port=7
  Constant2 : Constant  Value=2
  Constant6 : Constant  Value=6
  Embedded MATLAB Function : MATLAB Function  TreatAsAtomicUnit=on
  Gain1 : Gain  Gain=2
  Gain2 : Gain  Gain=180/pi
  Gain3 : Gain  Gain=pi/180
  Mux : Mux
  Phi050 DoE model : Subsystem
  q : Outport
  Q : Outport  Port=2
  wires:
  Gain2/1 -> Phi050 DoE model/4(VVT)
  Embedded MATLAB Function/2(Q) -> Q/1
  u/1 -> Embedded MATLAB Function/1(u)
  EGR/1 -> Phi050 DoE model/6(EGR)
  Gain1/1 -> Mux/3
  AF/1 -> Phi050 DoE model/5(AFR)
  VT/1 -> Gain2/1
  KL/1 -> Phi050 DoE model/2(KL)
  rps/1 -> Phi050 DoE model/1(N)
  Phi050 DoE model/1(Phi50) -> Gain1/1
  Constant2/1 -> Mux/2
  Constant6/1 -> Mux/1
  Mux/1 -> Embedded MATLAB Function/2(Web)
  SA/1 -> Phi050 DoE model/3(SA), Gain3/1
  Embedded MATLAB Function/1(q) -> q/1
  Gain3/1 -> Mux/4

== system benchmark_model_2/ENGINE/engine_s/cylinders/cyl4/cyl/knock_Integral/Subsystem1/Subsystem ==
  Tu : Inport
  Constant1 : Constant  Value=FR_C3
  Divide : Product  Inputs=/*
  Math Function1 : Math  SignedPower=on  SaturateOnIntegerOverflow=on
  Saturation : Saturate  UpperLimit=inf  LowerLimit=1.0e-5
  Out1 : Outport
  wires:
  Saturation/1 -> Divide/1
  Tu/1 -> Saturation/1
  Math Function1/1 -> Out1/1
  Divide/1 -> Math Function1/1
  Constant1/1 -> Divide/2

== system benchmark_model_2/ENGINE/engine_s/cylinders/cyl4/cyl/knock_Integral/Subsystem1/cal_unburned_temp ==
  Pc : Inport
  Tc : Inport  Port=2
  trg_inc : Inport  Port=3
  Constant : Constant  Value=1-1/Kex
  Divide3 : Product  Inputs=*/
  Divide4 : Product
  Math Function2 : Math  Operator=pow  SignedPower=on  SaturateOnIntegerOverflow=on
  Subsystem : Subsystem
  Tu : Outport
  wires:
  trg_inc/1 -> Subsystem/Trigger
  Pc/1 -> Divide3/1, Subsystem/1(Pc)
  Tc/1 -> Subsystem/2(Tc)
  Divide4/1 -> Tu/1
  Constant/1 -> Math Function2/2
  Subsystem/2(Tc_inc) -> Divide4/2
  Math Function2/1 -> Divide4/1
  Divide3/1 -> Math Function2/1
  Subsystem/1(Pc_inc) -> Divide3/2

== system benchmark_model_2/ENGINE/engine_s/cylinders/cyl1/cyl/frame/Init_cyl_gas/capture_cyl_state/burnt_compsition ==
  af : Inport
  mol_su : Inport  Port=2
  C : Constant  Value=WOM
  C1 : Constant  Value=WOM
  Dot Product : DotProduct  InputSameDT=on  OutDataTypeStr=Inherit: Inherit via internal rule
  Dot Product2 : DotProduct  InputSameDT=on  OutDataTypeStr=Inherit: Inherit via internal rule
  Mux : Mux  Inputs=7
  Product1 : Product  RndMeth=Zero
  Product2 : Product  Inputs=/*  RndMeth=Zero
  Saturation : Saturate  UpperLimit=22  LowerLimit=6
  Subsystem : Subsystem
  table_CO : Lookup  InputValues=AL  Table=[CO]*1.0e-2
  table_CO2 : Lookup  InputValues=AL  Table=[CO2]*1.0e-2
  table_H2 : Lookup  InputValues=AL  Table=[H2]*1.0e-2
  table_H2O : Lookup  InputValues=AL  Table=[H2O]*1.0e-2
  table_HC : Lookup  InputValues=AL  Table=[HC]*1.0e-6
  table_N2 : Lookup  InputValues=AL  Table=[N2]*1.0e-2
  table_O2 : Lookup  InputValues=AL  Table=[O2]*1.0e-2
  b_comp : Outport
  wires:
  Product2/1 -> Product1/2
  Product1/1 -> Subsystem/2(burnt)
  C/1 -> Dot Product/2
  table_HC/1 -> Mux/1
  table_N2/1 -> Mux/7
  table_CO2/1 -> Mux/2
  table_CO/1 -> Mux/3
  table_O2/1 -> Mux/4
  table_H2/1 -> Mux/5
  table_H2O/1 -> Mux/6
  af/1 -> Saturation/1, Subsystem/1(af)
  Mux/1 -> Product1/1, Dot Product/1
  Saturation/1 -> table_HC/1, table_CO2/1, table_CO/1, table_O2/1, table_H2/1, table_H2O/1, table_N2/1
  mol_su/1 -> Subsystem/3(unburnt), Dot Product2/2
  Subsystem/1(Out1) -> b_comp/1
  C1/1 -> Dot Product2/1
  Dot Product/1 -> Product2/1
  Dot Product2/1 -> Product2/2

== system benchmark_model_2/ENGINE/engine_s/cylinders/cyl1/cyl/frame/Init_cyl_gas/capture_cyl_state/cal_af ==
  cyl_gas : Inport
  Constant2 : Constant  Value=[0,MO2,MO2/2,MO2,0,MO2/2,MN2]
  Constant3 : Constant  Value=[1,1,1,0,0,0,0]
  Divide : Product  Inputs=/*
  Dot Product : DotProduct  InputSameDT=on  OutDataTypeStr=Inherit: Inherit via internal rule
  Dot Product2 : DotProduct  InputSameDT=on  OutDataTypeStr=Inherit: Inherit via internal rule
  Gain : Gain  Gain=MHC
  af : Outport
  wires:
  Gain/1 -> Divide/1
  Divide/1 -> af/1
  Constant3/1 -> Dot Product/2
  Dot Product/1 -> Gain/1
  cyl_gas/1 -> Dot Product/1, Dot Product2/1
  Dot Product2/1 -> Divide/2
  Constant2/1 -> Dot Product2/2

== system benchmark_model_2/ENGINE/engine_s/cylinders/cyl1/cyl/frame/ratio_burnt1/murnt_ratio/Phi050 DoE model ==
  N : Inport
  KL : Inport  Port=2
  SA : Inport  Port=3
  VVT : Inport  Port=4
  AFR : Inport  Port=5
  EGR : Inport  Port=6
  0 .. 1 : Saturate  UpperLimit=0.9  LowerLimit=0  ZeroCross=off
      settings: AttributesFormatString=%<LowerLimit> .. %<UpperLimit>
  Fcn : Fcn  Expr=C_EGR/(1-u)
  Product : Product
  Subsystem : Subsystem
  Phi50 : Outport
  wires:
  N/1 -> Subsystem/1(N)
  KL/1 -> Subsystem/2(KL)
  SA/1 -> Subsystem/3(SA)
  VVT/1 -> Subsystem/4(VVT)
  Subsystem/1(Phi50) -> Phi50/1
  EGR/1 -> 0 .. 1/1
  0 .. 1/1 -> Fcn/1
  AFR/1 -> Product/1
  Fcn/1 -> Product/2
  Product/1 -> Subsystem/5(AFR)

== system benchmark_model_2/ENGINE/engine_s/cylinders/cyl1/cyl/knock_Integral/Subsystem1/cal_unburned_temp/Subsystem ==
  Pc : Inport
  Tc : Inport  Port=2
  Trigger : TriggerPort  VariantControl=(inherit)
  Pc_inc : Outport  InitialOutput=[PR0]
  Tc_inc : Outport  Port=2  InitialOutput=[TM0]
  wires:
  Tc/1 -> Tc_inc/1
  Pc/1 -> Pc_inc/1

== system benchmark_model_2/ENGINE/engine_s/cylinders/cyl2/cyl/frame/Init_cyl_gas/capture_cyl_state/burnt_compsition ==
  af : Inport
  mol_su : Inport  Port=2
  C : Constant  Value=WOM
  C1 : Constant  Value=WOM
  Dot Product : DotProduct  InputSameDT=on  OutDataTypeStr=Inherit: Inherit via internal rule
  Dot Product2 : DotProduct  InputSameDT=on  OutDataTypeStr=Inherit: Inherit via internal rule
  Mux : Mux  Inputs=7
  Product1 : Product  RndMeth=Zero
  Product2 : Product  Inputs=/*  RndMeth=Zero
  Saturation : Saturate  UpperLimit=22  LowerLimit=6
  Subsystem : Subsystem
  table_CO : Lookup  InputValues=AL  Table=[CO]*1.0e-2
  table_CO2 : Lookup  InputValues=AL  Table=[CO2]*1.0e-2
  table_H2 : Lookup  InputValues=AL  Table=[H2]*1.0e-2
  table_H2O : Lookup  InputValues=AL  Table=[H2O]*1.0e-2
  table_HC : Lookup  InputValues=AL  Table=[HC]*1.0e-6
  table_N2 : Lookup  InputValues=AL  Table=[N2]*1.0e-2
  table_O2 : Lookup  InputValues=AL  Table=[O2]*1.0e-2
  b_comp : Outport
  wires:
  Dot Product2/1 -> Product2/2
  Dot Product/1 -> Product2/1
  C1/1 -> Dot Product2/1
  Subsystem/1(Out1) -> b_comp/1
  mol_su/1 -> Dot Product2/2, Subsystem/3(unburnt)
  Saturation/1 -> table_N2/1, table_H2O/1, table_H2/1, table_O2/1, table_CO/1, table_CO2/1, table_HC/1
  Mux/1 -> Dot Product/1, Product1/1
  af/1 -> Subsystem/1(af), Saturation/1
  table_H2O/1 -> Mux/6
  table_H2/1 -> Mux/5
  table_O2/1 -> Mux/4
  table_CO/1 -> Mux/3
  table_CO2/1 -> Mux/2
  table_N2/1 -> Mux/7
  table_HC/1 -> Mux/1
  C/1 -> Dot Product/2
  Product1/1 -> Subsystem/2(burnt)
  Product2/1 -> Product1/2

== system benchmark_model_2/ENGINE/engine_s/cylinders/cyl2/cyl/frame/Init_cyl_gas/capture_cyl_state/cal_af ==
  cyl_gas : Inport
  Constant2 : Constant  Value=[0,MO2,MO2/2,MO2,0,MO2/2,MN2]
  Constant3 : Constant  Value=[1,1,1,0,0,0,0]
  Divide : Product  Inputs=/*
  Dot Product : DotProduct  InputSameDT=on  OutDataTypeStr=Inherit: Inherit via internal rule
  Dot Product2 : DotProduct  InputSameDT=on  OutDataTypeStr=Inherit: Inherit via internal rule
  Gain : Gain  Gain=MHC
  af : Outport
  wires:
  Constant2/1 -> Dot Product2/2
  Dot Product2/1 -> Divide/2
  cyl_gas/1 -> Dot Product2/1, Dot Product/1
  Dot Product/1 -> Gain/1
  Constant3/1 -> Dot Product/2
  Divide/1 -> af/1
  Gain/1 -> Divide/1

== system benchmark_model_2/ENGINE/engine_s/cylinders/cyl2/cyl/frame/ratio_burnt1/murnt_ratio/Phi050 DoE model ==
  N : Inport
  KL : Inport  Port=2
  SA : Inport  Port=3
  VVT : Inport  Port=4
  AFR : Inport  Port=5
  EGR : Inport  Port=6
  0 .. 1 : Saturate  UpperLimit=0.9  LowerLimit=0  ZeroCross=off
      settings: AttributesFormatString=%<LowerLimit> .. %<UpperLimit>
  Fcn : Fcn  Expr=C_EGR/(1-u)
  Product : Product
  Subsystem : Subsystem
  Phi50 : Outport
  wires:
  Product/1 -> Subsystem/5(AFR)
  Fcn/1 -> Product/2
  AFR/1 -> Product/1
  0 .. 1/1 -> Fcn/1
  EGR/1 -> 0 .. 1/1
  Subsystem/1(Phi50) -> Phi50/1
  VVT/1 -> Subsystem/4(VVT)
  SA/1 -> Subsystem/3(SA)
  KL/1 -> Subsystem/2(KL)
  N/1 -> Subsystem/1(N)

== system benchmark_model_2/ENGINE/engine_s/cylinders/cyl2/cyl/knock_Integral/Subsystem1/cal_unburned_temp/Subsystem ==
  Pc : Inport
  Tc : Inport  Port=2
  Trigger : TriggerPort  VariantControl=(inherit)
  Pc_inc : Outport  InitialOutput=[PR0]
  Tc_inc : Outport  Port=2  InitialOutput=[TM0]
  wires:
  Pc/1 -> Pc_inc/1
  Tc/1 -> Tc_inc/1

== system benchmark_model_2/ENGINE/engine_s/cylinders/cyl3/cyl/frame/Init_cyl_gas/capture_cyl_state/burnt_compsition ==
  af : Inport
  mol_su : Inport  Port=2
  C : Constant  Value=WOM
  C1 : Constant  Value=WOM
  Dot Product : DotProduct  InputSameDT=on  OutDataTypeStr=Inherit: Inherit via internal rule
  Dot Product2 : DotProduct  InputSameDT=on  OutDataTypeStr=Inherit: Inherit via internal rule
  Mux : Mux  Inputs=7
  Product1 : Product  RndMeth=Zero
  Product2 : Product  Inputs=/*  RndMeth=Zero
  Saturation : Saturate  UpperLimit=22  LowerLimit=6
  Subsystem : Subsystem
  table_CO : Lookup  InputValues=AL  Table=[CO]*1.0e-2
  table_CO2 : Lookup  InputValues=AL  Table=[CO2]*1.0e-2
  table_H2 : Lookup  InputValues=AL  Table=[H2]*1.0e-2
  table_H2O : Lookup  InputValues=AL  Table=[H2O]*1.0e-2
  table_HC : Lookup  InputValues=AL  Table=[HC]*1.0e-6
  table_N2 : Lookup  InputValues=AL  Table=[N2]*1.0e-2
  table_O2 : Lookup  InputValues=AL  Table=[O2]*1.0e-2
  b_comp : Outport
  wires:
  Product2/1 -> Product1/2
  Product1/1 -> Subsystem/2(burnt)
  C/1 -> Dot Product/2
  table_HC/1 -> Mux/1
  table_N2/1 -> Mux/7
  table_CO2/1 -> Mux/2
  table_CO/1 -> Mux/3
  table_O2/1 -> Mux/4
  table_H2/1 -> Mux/5
  table_H2O/1 -> Mux/6
  af/1 -> Saturation/1, Subsystem/1(af)
  Mux/1 -> Product1/1, Dot Product/1
  Saturation/1 -> table_HC/1, table_CO2/1, table_CO/1, table_O2/1, table_H2/1, table_H2O/1, table_N2/1
  mol_su/1 -> Subsystem/3(unburnt), Dot Product2/2
  Subsystem/1(Out1) -> b_comp/1
  C1/1 -> Dot Product2/1
  Dot Product/1 -> Product2/1
  Dot Product2/1 -> Product2/2

== system benchmark_model_2/ENGINE/engine_s/cylinders/cyl3/cyl/frame/Init_cyl_gas/capture_cyl_state/cal_af ==
  cyl_gas : Inport
  Constant2 : Constant  Value=[0,MO2,MO2/2,MO2,0,MO2/2,MN2]
  Constant3 : Constant  Value=[1,1,1,0,0,0,0]
  Divide : Product  Inputs=/*
  Dot Product : DotProduct  InputSameDT=on  OutDataTypeStr=Inherit: Inherit via internal rule
  Dot Product2 : DotProduct  InputSameDT=on  OutDataTypeStr=Inherit: Inherit via internal rule
  Gain : Gain  Gain=MHC
  af : Outport
  wires:
  Gain/1 -> Divide/1
  Divide/1 -> af/1
  Constant3/1 -> Dot Product/2
  Dot Product/1 -> Gain/1
  cyl_gas/1 -> Dot Product/1, Dot Product2/1
  Dot Product2/1 -> Divide/2
  Constant2/1 -> Dot Product2/2

== system benchmark_model_2/ENGINE/engine_s/cylinders/cyl3/cyl/frame/ratio_burnt1/murnt_ratio/Phi050 DoE model ==
  N : Inport
  KL : Inport  Port=2
  SA : Inport  Port=3
  VVT : Inport  Port=4
  AFR : Inport  Port=5
  EGR : Inport  Port=6
  0 .. 1 : Saturate  UpperLimit=0.9  LowerLimit=0  ZeroCross=off
      settings: AttributesFormatString=%<LowerLimit> .. %<UpperLimit>
  Fcn : Fcn  Expr=C_EGR/(1-u)
  Product : Product
  Subsystem : Subsystem
  Phi50 : Outport
  wires:
  N/1 -> Subsystem/1(N)
  KL/1 -> Subsystem/2(KL)
  SA/1 -> Subsystem/3(SA)
  VVT/1 -> Subsystem/4(VVT)
  Subsystem/1(Phi50) -> Phi50/1
  EGR/1 -> 0 .. 1/1
  0 .. 1/1 -> Fcn/1
  AFR/1 -> Product/1
  Fcn/1 -> Product/2
  Product/1 -> Subsystem/5(AFR)

== system benchmark_model_2/ENGINE/engine_s/cylinders/cyl3/cyl/knock_Integral/Subsystem1/cal_unburned_temp/Subsystem ==
  Pc : Inport
  Tc : Inport  Port=2
  Trigger : TriggerPort  VariantControl=(inherit)
  Pc_inc : Outport  InitialOutput=[PR0]
  Tc_inc : Outport  Port=2  InitialOutput=[TM0]
  wires:
  Tc/1 -> Tc_inc/1
  Pc/1 -> Pc_inc/1
